simulink model "xy_graph"  (R2021a)
settings: Solver=VariableStepAuto  StartTime=0.0  StopTime=10.0  RelTol=1e-3
libraries: simulink x2
settings Model: Creator=Aula  LastModifiedBy=Aula

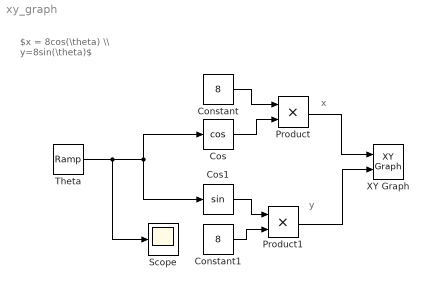
== system xy_graph ==
  note: y
  note: x
  note: $x = 8cos(\theta) \\ y=8sin(\theta)$
  Constant : Constant  Value=8
  Constant1 : Constant  Value=8
  Cos : Trigonometry  Operator=cos
  Cos1 : Trigonometry
  Product : Product
  Product1 : Product
  Scope : Scope
  Theta : simulink/Sources/Ramp  slope=1  start=0  InitialOutput=0
  XY Graph : simulink/Sinks/XY Graph  xmin=-20  xmax=20  ymin=-20  ymax=20  st=-1
  wires:
  Theta/1 -> Scope/1, Cos/1, Cos1/1
  Constant/1 -> Product/1
  Cos/1 -> Product/2
  Cos1/1 -> Product1/1
  Constant1/1 -> Product1/2
  Product/1 -> XY Graph/1
  Product1/1 -> XY Graph/2
